simulink library "my_math_ops"  (R2021b)
settings: Solver=VariableStepAuto  StartTime=0.0  StopTime=10.0  RelTol=1e-3
settings Model: Creator=Davide  LastModifiedBy=Davide
settings SolverCC: AlgebraicLoopSolver=TrustRegion
settings DebuggingCC: SFMachineParentedDataDiag=warning

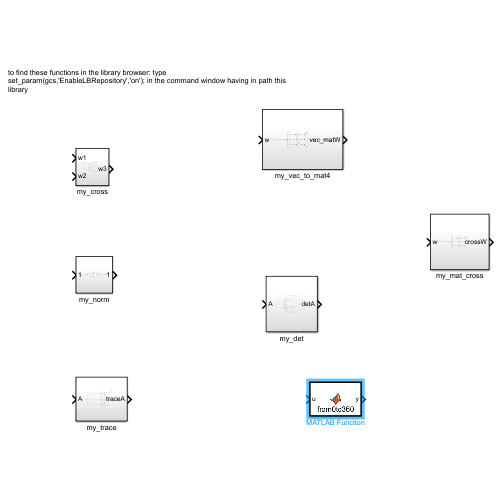
[thumbnail: Simulink's stored preview of the top-level diagram]
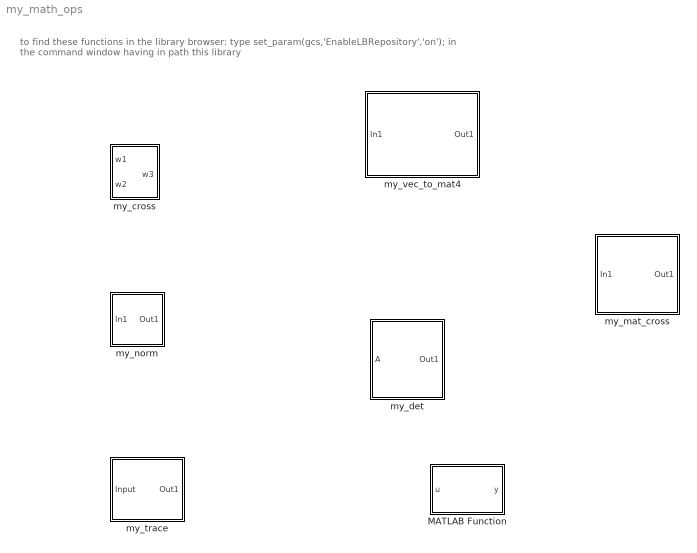
== system my_math_ops ==
  note: to find these functions in the library browser: type set_param(gcs,'EnableLBRepository','on'); in the command window having in path this library
  MATLAB Function : MATLAB Function  TreatAsAtomicUnit=on
  my_cross : Subsystem
  my_det : Subsystem
  my_mat_cross : Subsystem
  my_norm : Subsystem
  my_trace : Subsystem
  my_vec_to_mat4 : Subsystem

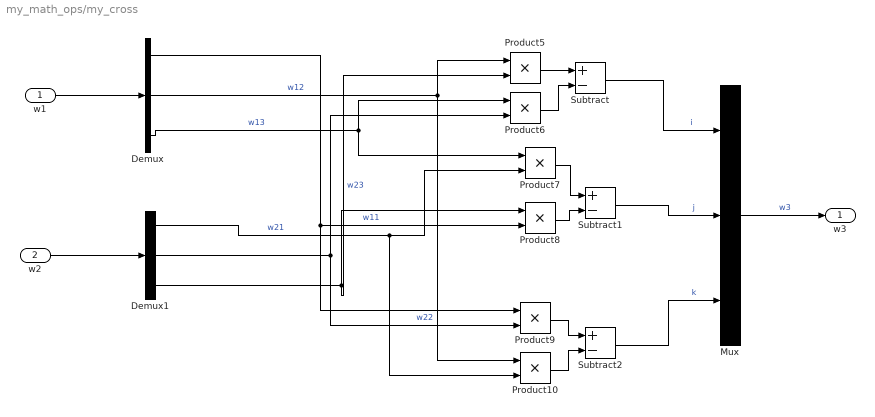
== system my_math_ops/my_cross ==
  w1 : Inport
  w2 : Inport  Port=2
  Demux : Demux  Outputs=3
  Demux1 : Demux  Outputs=3
  Mux : Mux  Inputs=3
  Product{5..10} (6 alike) : Product
  Subtract : Sum  Inputs=+-
  Subtract1 : Sum  Inputs=+-
  Subtract2 : Sum  Inputs=+-
  w3 : Outport
  wires:
  Subtract1/1 -> Mux/2  "j"
  Product6/1 -> Subtract/2
  Demux1/3 -> Product5/2, Product8/1  "w23"
  Demux/1 -> Product9/1, Product8/2  "w11"
  Demux/3 -> Product7/1, Product6/1  "w13"
  Product5/1 -> Subtract/1
  Demux1/1 -> Product10/2, Product7/2  "w21"
  Product9/1 -> Subtract2/1
  Demux1/2 -> Product9/2, Product6/2  "w22"
  Demux/2 -> Product5/1, Product10/1  "w12"
  Subtract/1 -> Mux/1  "i"
  w2/1 -> Demux1/1
  Product10/1 -> Subtract2/2
  Product7/1 -> Subtract1/1
  Product8/1 -> Subtract1/2
  Subtract2/1 -> Mux/3  "k"
  w1/1 -> Demux/1
  Mux/1 -> w3/1  "w3"

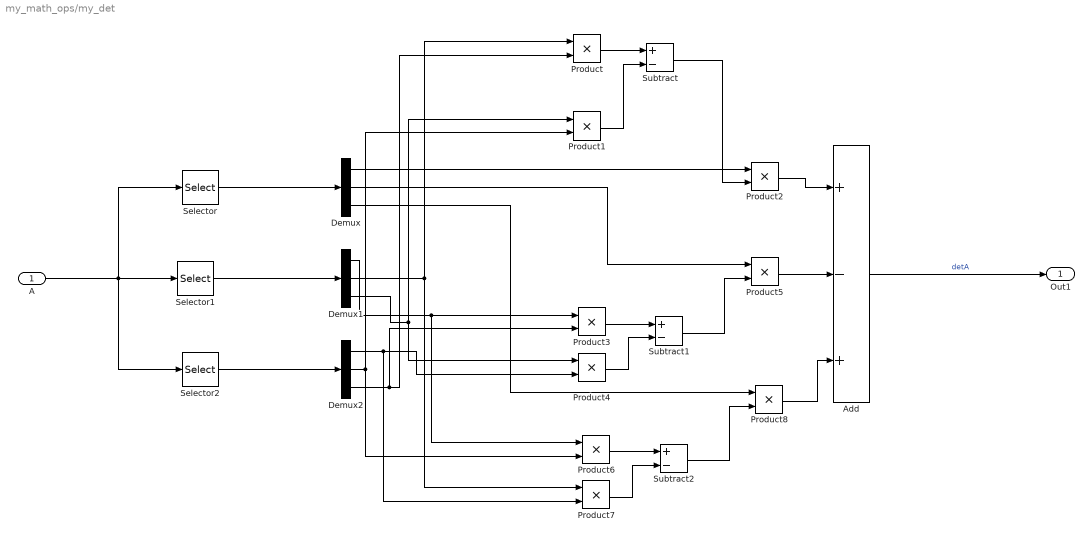
== system my_math_ops/my_det ==
  A : Inport
  Add : Sum  Inputs=+-+
  Demux : Demux  Outputs=3
  Demux1 : Demux  Outputs=3
  Demux2 : Demux  Outputs=3
  Product{,1..8} (9 alike) : Product
  Selector : Selector  NumberOfDimensions=2  InputPortWidth=3  IndexOptions=Index vector (dialog),Select all  Indices=1,1  OutputSizes=1,1
  Selector1 : Selector  NumberOfDimensions=2  InputPortWidth=3  IndexOptions=Index vector (dialog),Select all  Indices=2,1  OutputSizes=1,1
  Selector2 : Selector  NumberOfDimensions=2  InputPortWidth=3  IndexOptions=Index vector (dialog),Select all  Indices=3,1  OutputSizes=1,1
  Subtract : Sum  Inputs=+-
  Subtract1 : Sum  Inputs=+-
  Subtract2 : Sum  Inputs=+-
  Out1 : Outport
  wires:
  Subtract2/1 -> Product8/2
  Product8/1 -> Add/3
  Demux/1 -> Product2/1
  Demux1/3 -> Product4/1, Product1/1
  Selector2/1 -> Demux2/1
  Demux2/3 -> Product3/2, Product/2
  Product1/1 -> Subtract/2
  Subtract1/1 -> Product5/2
  Product5/1 -> Add/2
  Product6/1 -> Subtract2/1
  Demux1/2 -> Product7/1, Product/1
  Product7/1 -> Subtract2/2
  Product2/1 -> Add/1
  Selector1/1 -> Demux1/1
  Selector/1 -> Demux/1
  A/1 -> Selector/1, Selector2/1, Selector1/1
  Demux/3 -> Product8/1
  Product3/1 -> Subtract1/1
  Product/1 -> Subtract/1
  Subtract/1 -> Product2/2
  Demux2/2 -> Product6/2, Product1/2
  Product4/1 -> Subtract1/2
  Demux2/1 -> Product7/2, Product4/2
  Demux1/1 -> Product6/1, Product3/1
  Demux/2 -> Product5/1
  Add/1 -> Out1/1  "detA"

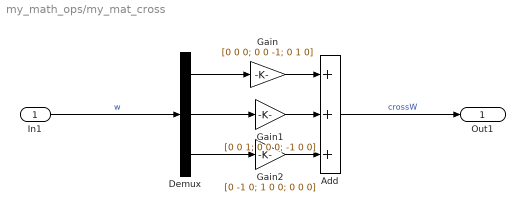
== system my_math_ops/my_mat_cross ==
  In1 : Inport
  Add : Sum  Inputs=+++
  Demux : Demux  Outputs=3
  Gain : Gain  Gain=[0 0 0; 0 0 -1; 0 1 0]
  Gain1 : Gain  Gain=[0 0 1; 0 0 0; -1 0 0]
  Gain2 : Gain  Gain=[0 -1 0; 1 0 0; 0 0 0]
  Out1 : Outport
  wires:
  In1/1 -> Demux/1  "w"
  Gain1/1 -> Add/2
  Gain2/1 -> Add/3
  Demux/2 -> Gain1/1
  Add/1 -> Out1/1  "crossW"
  Gain/1 -> Add/1
  Demux/3 -> Gain2/1
  Demux/1 -> Gain/1

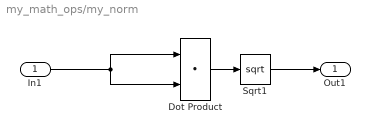
== system my_math_ops/my_norm ==
  In1 : Inport
  Dot Product : DotProduct  InputSameDT=on  OutDataTypeStr=Inherit: Inherit via internal rule
  Sqrt1 : Sqrt  SaturateOnIntegerOverflow=on
  Out1 : Outport
  wires:
  Dot Product/1 -> Sqrt1/1
  In1/1 -> Dot Product/2, Dot Product/1
  Sqrt1/1 -> Out1/1

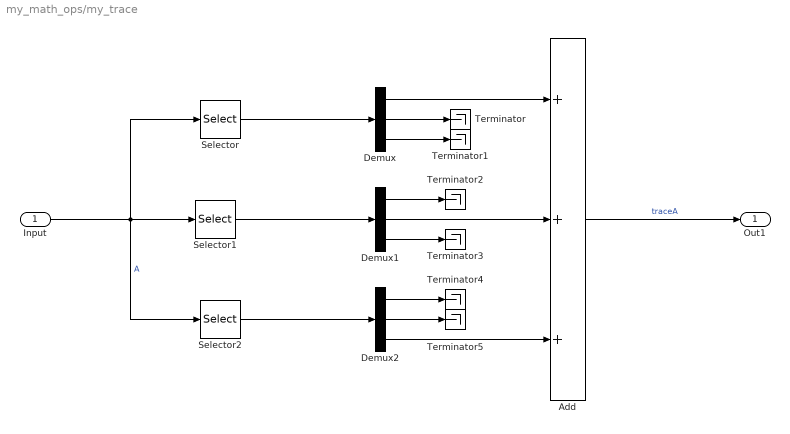
== system my_math_ops/my_trace ==
  Input : Inport
  Add : Sum  Inputs=+++
  Demux : Demux  Outputs=3
  Demux1 : Demux  Outputs=3
  Demux2 : Demux  Outputs=3
  Selector : Selector  NumberOfDimensions=2  InputPortWidth=3  IndexOptions=Index vector (dialog),Select all  Indices=1,1  OutputSizes=1,1
  Selector1 : Selector  NumberOfDimensions=2  InputPortWidth=3  IndexOptions=Index vector (dialog),Select all  Indices=2,1  OutputSizes=1,1
  Selector2 : Selector  NumberOfDimensions=2  InputPortWidth=3  IndexOptions=Index vector (dialog),Select all  Indices=3,1  OutputSizes=1,1
  Terminator{,1..5} (6 alike) : Terminator
  Out1 : Outport
  wires:
  Demux2/1 -> Terminator4/1
  Selector2/1 -> Demux2/1
  Selector/1 -> Demux/1
  Demux/2 -> Terminator/1
  Demux1/1 -> Terminator2/1
  Demux2/2 -> Terminator5/1
  Demux1/3 -> Terminator3/1
  Selector1/1 -> Demux1/1
  Demux2/3 -> Add/3
  Input/1 -> Selector/1, Selector2/1, Selector1/1  "A"
  Demux/1 -> Add/1
  Demux/3 -> Terminator1/1
  Demux1/2 -> Add/2
  Add/1 -> Out1/1  "traceA"

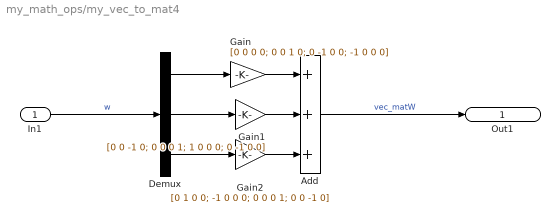
== system my_math_ops/my_vec_to_mat4 ==
  In1 : Inport
  Add : Sum  Inputs=+++
  Demux : Demux  Outputs=3
  Gain : Gain  Gain=[0 0 0 0; 0 0 1 0; 0 -1 0 0; -1 0 0 0]
  Gain1 : Gain  Gain=[0 0 -1 0; 0 0 0 1; 1 0 0 0; 0 -1 0 0]
  Gain2 : Gain  Gain=[0 1 0 0; -1 0 0 0; 0 0 0 1; 0 0 -1 0]
  Out1 : Outport
  wires:
  In1/1 -> Demux/1  "w"
  Gain1/1 -> Add/2
  Gain2/1 -> Add/3
  Demux/2 -> Gain1/1
  Add/1 -> Out1/1  "vec_matW"
  Gain/1 -> Add/1
  Demux/3 -> Gain2/1
  Demux/1 -> Gain/1

== matlab function my_math_ops/MATLAB Function ==
  data: u input; y output
function y = from0to360(u)
while u>360
    u=u-360;
end
while u<0
    u=u+360;
end
y = u;
